simulink model "bikesim_magic_formula"  (R2026a)
settings: Solver=ode45  MaxStep=1E-03
InitFcn:
  | moto_init;
values from neighbouring files (symbols this model uses):
  p = motoParameters    [bikeSimToMotoParameters.m]    (also in moto_init.m = bikeSimToPrydeV2Parameters(bs,130/3.6); moto_trim_test.m = P{idx_vx}; steadyTurningTrimEqns.m = in3(41,:); steadyTurningTrimJac.m = in3(41,:))
  pr = table2struct(rt.Pacejka)    [moto_init.m]    (also in moto_trim_test.m = fpacejka(bs.RearTire.Pacejka))
libraries: simulink x2, simulink_extras x1
(part 1 of 2)
settings Model: Creator=marti  LastModifiedBy=marti

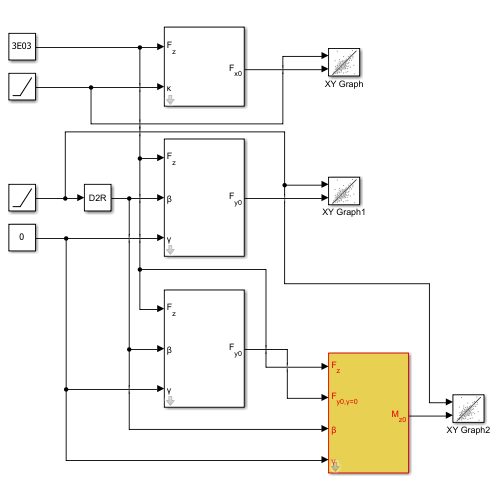
[thumbnail: Simulink's stored preview of the top-level diagram]
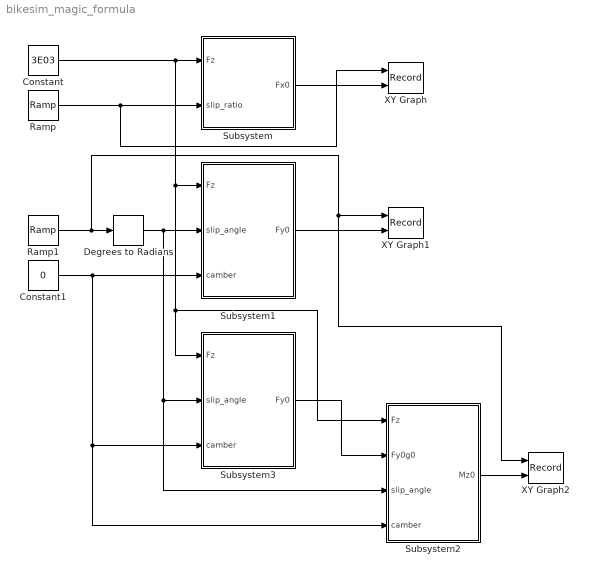
== system bikesim_magic_formula ==
  Constant : Constant  Value=3E03
  Constant1 : Constant  Value=0
  Degrees to Radians : simulink_extras/Transformations/Degrees to Radians
  Ramp : simulink/Sources/Ramp  slope=0.18  start=0  InitialOutput=-0.9
  Ramp1 : simulink/Sources/Ramp  slope=6  start=0  InitialOutput=-30
  Subsystem : Subsystem  mask(Longitudinal force (pure slip)){Fz0=pr.fz0, Cx=pr.pcx1, pdx1=pr.pdx1, pdx2=pr.pdx2, pex1=pr.pex1, pex2=pr.pex2, pex3=pr.pex3, pkx1=pr.pkx1, pkx2=pr.pkx2, pkx3=pr.pkx3}
      mask prompts: Fz0 "F_z0"; Cx "C_x"; pdx1 "p_Dx1"; pdx2 "p_Dx2"; pex1 "p_Ex1"; pex2 "p_Ex2"; pex3 "p_Ex3"; pkx1 "p_Kx1"; pkx2 "p_Kx2"; pkx3 "p_Kx3"
      mask help: Implements (11)-(16) from the BikeSim 2017.1 Tire_Models documentation.
      mask TypeOptions Fz0: Normal force ratio/Fz0
      mask TypeOptions Cx: Magic formula/Cx | Stiffness factor/Cx
      mask TypeOptions pdx1: Peak factor/pdx1
      mask TypeOptions pdx2: Peak factor/pdx2
      mask TypeOptions pex1: Curvature factor/pex1
      mask TypeOptions pex2: Curvature factor/pex2
      mask TypeOptions pex3: Curvature factor/pex3
      mask TypeOptions pkx1: Stiffness factor/pkx1
      mask TypeOptions pkx2: Stiffness factor/pkx2
      mask TypeOptions pkx3: Stiffness factor/pkx3
      mask Display:
      | port_label('input', 1, 'F_z','Interpreter','tex');
      | port_label('input', 2, '\kappa','Interpreter','tex');
      | port_label('output', 1, 'F_{x0}','Interpreter','tex');
  Subsystem1 : Subsystem  mask{Fz0=pr.fz0, Cy=pr.pcy1, Cg=pr.pcy2, pdy1=pr.pdy1, pdy2=pr.pdy2, pdy3=pr.pdy3, pey1=pr.pey1, pey2=pr.pey2, pey4=pr.pey4, Eg=pr.pey5, pky1=pr.pky1, pky2=pr.pky2, pky3=pr.pky3, pky4=pr.pky4, pky5=pr.pky5, pky6=pr.pky6, pky7=pr.pky7}
      mask prompts: Fz0 "F_z0"; Cy "C_y"; Cg "C_g"; pdy1 "p_Dy1"; pdy2 "p_Dy2"; pdy3 "p_Dy3"; pey1 "p_Ey1"; pey2 "p_Ey2"; pey4 "p_Ey4"; Eg "E_g"; pky1 "p_Ky1"; pky2 "p_Ky2"; pky3 "p_Ky3"; pky4 "p_Ky4"; pky5 "p_Ky5"; pky6 "p_Ky6"; pky7 "p_Ky7"
      mask TypeOptions Fz0: Normal force ratio/Fz0 | Lateral force (slip)/Fz0
      mask TypeOptions Cy: Lateral force (slip)/Cy
      mask TypeOptions Cg: Lateral force (camber)/Cg
      mask TypeOptions pdy1: Peak factor/pdy1
      mask TypeOptions pdy2: Peak factor/pdy2
      mask TypeOptions pdy3: Peak factor/pdy3
      mask TypeOptions pey1: Lateral force (slip)/pey1
      mask TypeOptions pey2: Lateral force (slip)/pey2
      mask TypeOptions pey4: Lateral force (slip)/pey4
      mask TypeOptions Eg: Lateral force (camber)/Eg
      mask TypeOptions pky1: Lateral force (slip)/pky1
      mask TypeOptions pky2: Lateral force (slip)/pky2
      mask TypeOptions pky3: Lateral force (slip)/pky3
      mask TypeOptions pky4: Lateral force (slip)/pky4
      mask TypeOptions pky5: Lateral force (slip)/pky5
      mask TypeOptions pky6: Lateral force (camber)/pky6
      mask TypeOptions pky7: Lateral force (camber)/pky7
      mask Display:
      | port_label('input', 1, 'F_z','Interpreter','tex');
      | port_label('input', 2, '\beta','Interpreter','tex');
      | port_label('input', 3, '\gamma','Interpreter','tex');
      | port_label('output', 1, 'F_{y0}','Interpreter','tex');
  Subsystem2 : Subsystem  mask{R0=p.tr, Cy=pr.pcy1, Ct=pr.qcz1, Fz0=pr.fz0, qbz1=pr.qbz1, qbz2=pr.qbz2, qbz5=pr.qbz5, qbz6=pr.qbz6, qbz9=pr.qbz9, qbz10=pr.qbz10, qdz1=pr.qdz1, qdz2=pr.qdz2, qdz3=pr.qdz3, qdz4=pr.qdz4, qdz8=pr.qdz8, qdz9=pr.qdz9, qdz10=pr.qdz10, qdz11=pr.qdz11, qez1=pr.qez1, qez2=pr.qez2, qez5=pr.qez5, qhz3=pr.qhz3, qhz4=pr.qhz4}
      mask prompts: R0 "R_0"; Cy "C_y"; Ct "C_t"; Fz0 "F_z0"; qbz1 "q_Bz1"; qbz2 "q_Bz2"; qbz5 "q_Bz5"; qbz6 "q_Bz6"; qbz9 "q_Bz9"; qbz10 "q_Bz10"; qdz1 "q_Dz1"; qdz2 "q_Dz2"; qdz3 "q_Dz3"; qdz4 "q_Dz4"; qdz8 "q_Dz8"; qdz9 "q_Dz9"; qdz10 "q_Dz10"; qdz11 "q_Dz11"; qez1 "q_Ez1"; qez2 "q_Ez2"; qez5 "q_Ez5"; qhz3 "q_Hz3"; qhz4 "q_Hz4"
      mask TypeOptions R0: Aligning moment (residual)/R0 | Aligning moment (trail)/R0
      mask TypeOptions Cy: Aligning moment (residual)/Cy
      mask TypeOptions Ct: Aligning moment (trail)/Ct
      mask TypeOptions Fz0: Aligning moment (trail)/Fz0
      mask TypeOptions qbz1: Aligning moment (trail)/qbz1
      mask TypeOptions qbz2: Aligning moment (trail)/qbz2
      mask TypeOptions qbz5: Aligning moment (trail)/qbz5
      mask TypeOptions qbz6: Aligning moment (trail)/qbz6
      mask TypeOptions qbz9: Aligning moment (residual)/qbz9
      mask TypeOptions qbz10: Aligning moment (residual)/qbz10
      mask TypeOptions qdz1: Aligning moment (trail)/qdz1
      mask TypeOptions qdz2: Aligning moment (trail)/qdz2
      mask TypeOptions qdz3: Aligning moment (trail)/qdz3
      mask TypeOptions qdz4: Aligning moment (trail)/qdz4
      mask TypeOptions qdz8: Aligning moment (residual)/qdz8
      mask TypeOptions qdz9: Aligning moment (residual)/qdz9
      mask TypeOptions qdz10: Aligning moment (residual)/qdz10
      mask TypeOptions qdz11: Aligning moment (residual)/qdz11
      mask TypeOptions qez1: Aligning moment (trail)/qez1
      mask TypeOptions qez2: Aligning moment (trail)/qez2
      mask TypeOptions qez5: Aligning moment (trail)/qez5
      mask TypeOptions qhz3: Aligning moment (residual)/qhz3
      mask TypeOptions qhz4: Aligning moment (residual)/qhz4
      mask Display:
      | port_label('input', 1, 'F_z','Interpreter','tex');
      | port_label('input', 2, 'F_{y0,\gamma=0}','Interpreter','tex');
      | port_label('input', 3, '\beta','Interpreter','tex');
      | port_label('input', 4, '\gamma','Interpreter','tex');
      | port_label('output', 1, 'M_{z0}','Interpreter','tex');
  Subsystem3 : Subsystem  mask{Fz0=pr.fz0, Cy=pr.pcy1, Cg=pr.pcy2, pdy1=pr.pdy1, pdy2=pr.pdy2, pdy3=pr.pdy3, pey1=pr.pey1, pey2=pr.pey2, pey4=pr.pey4, Eg=pr.pey5, pky1=pr.pky1, pky2=pr.pky2, pky3=pr.pky3, pky4=pr.pky4, pky5=pr.pky5, pky6=pr.pky6, pky7=pr.pky7}
      mask prompts: Fz0 "F_z0"; Cy "C_y"; Cg "C_g"; pdy1 "p_Dy1"; pdy2 "p_Dy2"; pdy3 "p_Dy3"; pey1 "p_Ey1"; pey2 "p_Ey2"; pey4 "p_Ey4"; Eg "E_g"; pky1 "p_Ky1"; pky2 "p_Ky2"; pky3 "p_Ky3"; pky4 "p_Ky4"; pky5 "p_Ky5"; pky6 "p_Ky6"; pky7 "p_Ky7"
      mask TypeOptions Fz0: Normal force ratio/Fz0 | Lateral force (slip)/Fz0
      mask TypeOptions Cy: Lateral force (slip)/Cy
      mask TypeOptions Cg: Lateral force (camber)/Cg
      mask TypeOptions pdy1: Peak factor/pdy1
      mask TypeOptions pdy2: Peak factor/pdy2
      mask TypeOptions pdy3: Peak factor/pdy3
      mask TypeOptions pey1: Lateral force (slip)/pey1
      mask TypeOptions pey2: Lateral force (slip)/pey2
      mask TypeOptions pey4: Lateral force (slip)/pey4
      mask TypeOptions Eg: Lateral force (camber)/Eg
      mask TypeOptions pky1: Lateral force (slip)/pky1
      mask TypeOptions pky2: Lateral force (slip)/pky2
      mask TypeOptions pky3: Lateral force (slip)/pky3
      mask TypeOptions pky4: Lateral force (slip)/pky4
      mask TypeOptions pky5: Lateral force (slip)/pky5
      mask TypeOptions pky6: Lateral force (camber)/pky6
      mask TypeOptions pky7: Lateral force (camber)/pky7
      mask Display:
      | port_label('input', 1, 'F_z','Interpreter','tex');
      | port_label('input', 2, '\beta','Interpreter','tex');
      | port_label('input', 3, '\gamma','Interpreter','tex');
      | port_label('output', 1, 'F_{y0}','Interpreter','tex');
  XY Graph : Record  NumPorts=2.0  FileSettingsInternal="{\"entries\":[{\"content\":{\"excelSettings\":{\"content\":{},\"type\":\"Streamout.ExcelSettings\"},\"parquetSettings\":{\"content\":{},\"type\":\"Streamout.ParquetSettings\"}},\"type\":\"Streamout.FileSettingStorage\",\"uuid\":\"\"}],\"packageUris\":[\"http:\\/\\/schema.mathworks.com\\/mf0\\/streamout_blocks\\/R2020a\"],\"version\":\"1.0\"}"  FrameSettings=[0, 0]  Layout=[1 1]  SignalsInternal="{\"entries\":[{\"content\":{\"signals\":[{\"content\":{\"blockPath\":[],\"dimensions\":[1],\"domain\":\"\",\"lineColor\":\"#a2142f\",\"plots\":[ 1 ],\"port\":1,\"sid\":[\"\"],\"signalID\":1,\"signalName\":\"Ramp\"},\"type\":\"RecordBlkView.Signal\",\"uuid\":\"\"},{\"content\":{\"blockPath\":[],\"dimensions\":[1],\"domain\":\"\",\"lineColor\":\"#139fff\",\"plots\":[ 1 ],\"port\":2,\"sid\":[\"\"],\"signalID\":2,\"signalName\":\"Subsystem\"},\"type\":\"RecordBlkView.Signal\",\"uuid\":\"\"}]},\"type\":\"RecordBlkView.InputSignals\",\"uuid\":\"\"}],\"packageUris\":[\"http:\\/\\/schema.mathworks.com\\/mf0\\/streamout_blocks\\/R2020a\"],\"version\":\"1.0\"}"  VisualizationBindings="{\"xyplotplugin\":{\"info\":[{\"series\":[{\"bindingParametersList\":[{\"parameter\":\"X-Axis\",\"signalID\":1,\"signalName\":\"Ramp\"},{\"parameter\":\"Y-Axis\",\"signalID\":2,\"signalName\":\"Subsystem\"}],\"seriesID\":0}],\"subplotID\":1}]}}"  CompatibilityTag=XY
  XY Graph1 : Record  NumPorts=2.0  FileSettingsInternal="{\"entries\":[{\"content\":{\"excelSettings\":{\"content\":{},\"type\":\"Streamout.ExcelSettings\"},\"parquetSettings\":{\"content\":{},\"type\":\"Streamout.ParquetSettings\"}},\"type\":\"Streamout.FileSettingStorage\",\"uuid\":\"\"}],\"packageUris\":[\"http:\\/\\/schema.mathworks.com\\/mf0\\/streamout_blocks\\/R2020a\"],\"version\":\"1.0\"}"  FrameSettings=[0, 0]  Layout=[1 1]  SignalsInternal="{\"entries\":[{\"content\":{\"signals\":[{\"content\":{\"blockPath\":[],\"dimensions\":[1],\"domain\":\"\",\"lineColor\":\"#a2142f\",\"plots\":[ 1 ],\"port\":1,\"sid\":[\"\"],\"signalID\":1,\"signalName\":\"Ramp1\"},\"type\":\"RecordBlkView.Signal\",\"uuid\":\"\"},{\"content\":{\"blockPath\":[],\"dimensions\":[1],\"domain\":\"\",\"lineColor\":\"#139fff\",\"plots\":[ 1 ],\"port\":2,\"sid\":[\"\"],\"signalID\":2,\"signalName\":\"Subsystem1\"},\"type\":\"RecordBlkView.Signal\",\"uuid\":\"\"}]},\"type\":\"RecordBlkView.InputSignals\",\"uuid\":\"\"}],\"packageUris\":[\"http:\\/\\/schema.mathworks.com\\/mf0\\/streamout_blocks\\/R2020a\"],\"version\":\"1.0\"}"  VisualizationBindings="{\"xyplotplugin\":{\"info\":[{\"series\":[{\"bindingParametersList\":[{\"parameter\":\"X-Axis\",\"signalID\":1,\"signalName\":\"Ramp1\"},{\"parameter\":\"Y-Axis\",\"signalID\":2,\"signalName\":\"Subsystem1\"}],\"seriesID\":0}],\"subplotID\":1}]}}"  CompatibilityTag=XY
  XY Graph2 : Record  NumPorts=2.0  FileSettingsInternal="{\"entries\":[{\"content\":{\"excelSettings\":{\"content\":{},\"type\":\"Streamout.ExcelSettings\"},\"parquetSettings\":{\"content\":{},\"type\":\"Streamout.ParquetSettings\"}},\"type\":\"Streamout.FileSettingStorage\",\"uuid\":\"\"}],\"packageUris\":[\"http:\\/\\/schema.mathworks.com\\/mf0\\/streamout_blocks\\/R2020a\"],\"version\":\"1.0\"}"  FrameSettings=[0, 0]  Layout=[1 1]  SignalsInternal="{\"entries\":[{\"content\":{\"signals\":[{\"content\":{\"blockPath\":[],\"dimensions\":[1],\"domain\":\"\",\"lineColor\":\"#a2142f\",\"plots\":[ 1 ],\"port\":1,\"signalID\":1,\"signalName\":\"XY Graph:1\"},\"type\":\"RecordBlkView.Signal\",\"uuid\":\"\"},{\"content\":{\"blockPath\":[],\"dimensions\":[1],\"domain\":\"\",\"lineColor\":\"#139fff\",\"plots\":[ 1 ],\"port\":2,\"signalID\":2,\"signalName\":\"XY Graph:2\"},\"type\":\"RecordBlkView.Signal\",\"uuid\":\"\"}]},\"type\":\"RecordBlkView.InputSignals\",\"uuid\":\"\"}],\"packageUris\":[\"http:\\/\\/schema.mathworks.com\\/mf0\\/streamout_blocks\\/R2020a\"],\"version\":\"1.0\"}"  VisualizationBindings="{\"xyplotplugin\":{\"info\":[{\"series\":[{\"bindingParametersList\":[{\"parameter\":\"X-Axis\",\"signalID\":1,\"signalName\":\"XY Graph:1\"},{\"parameter\":\"Y-Axis\",\"signalID\":2,\"signalName\":\"XY Graph:2\"}],\"seriesID\":0}],\"subplotID\":1}]}}"  CompatibilityTag=XY
  wires:
  Constant/1 -> Subsystem3/1(Fz), Subsystem2/1(Fz), Subsystem1/1(Fz), Subsystem/1(Fz)
  Ramp/1 -> XY Graph/1, Subsystem/2(slip_ratio)
  Ramp1/1 -> XY Graph2/1, XY Graph1/1, Degrees to Radians/1
  Constant1/1 -> Subsystem2/4(camber), Subsystem3/3(camber), Subsystem1/3(camber)
  Degrees to Radians/1 -> Subsystem2/3(slip_angle), Subsystem3/2(slip_angle), Subsystem1/2(slip_angle)
  Subsystem/1(Fx0) -> XY Graph/2
  Subsystem1/1(Fy0) -> XY Graph1/2
  Subsystem3/1(Fy0) -> Subsystem2/2(Fy0g0)
  Subsystem2/1(Mz0) -> XY Graph2/2

== system bikesim_magic_formula/Subsystem ==
  Fz : Inport
  slip_ratio : Inport  Port=2
  Curvature factor : Subsystem  mask(Curvature factor: longitudinal){pex1=pex1, pex2=pex2, pex3=pex3}
      mask prompts: pex1 "p_Ex1"; pex2 "p_Ex2"; pex3 "p_Ex3"
      mask help: Implements (14) from the BikeSim 2017.1 Tire_Models documentation.
      mask Display:
      | port_label('input', 1, 'd_{fz}','Interpreter','tex');
      | port_label('input', 2, '\kappa','Interpreter','tex');
      | port_label('output', 1, 'E_x','Interpreter','tex');
      | disp('(p_{Ex1} + p_{Ex2}\cdotdf_z + p_{Ex3}\cdotdf_{z}^{2})\cdot(1 - sgn(\kappa))','Interpreter','tex');
  Magic formula : Subsystem  mask(Magic formula: longitudinal (pure slip)){Cx=Cx}
      mask prompts: Cx "C_x"
      mask help: Implements (12) from the BikeSim 2017.1 Tire_Models documentation.
      mask TypeOptions Cx: Cx/Gain
      mask Display:
      | port_label('input', 1, 'D_x','Interpreter','tex');
      | port_label('input', 2, 'E_x','Interpreter','tex');
      | port_label('input', 3, 'B_x','Interpreter','tex');
      | port_label('input', 4, '\kappa','Interpreter','tex');
      | port_label('output', 1, 'F_{x0}','Interpreter','tex');
      | disp('D_x\cdotsin(C_x\cdotatan(B_x\cdot\kappa - E_x\cdot(B_x\cdot\kappa - atan(B_x\cdot\kappa))))','Interpreter','tex');
  Normal force ratio : Subsystem  mask(Normal force ratio){Fz0=Fz0}
      mask prompts: Fz0 "Nominal normal force"
      mask help: Implements (11) from the BikeSim 2017.1 Tire_models help documentation.
      mask TypeOptions Fz0: Fz0/Value
      mask Display:
      | port_label('output', 1, 'df_z','interpreter','tex');
      | port_label('input', 1, 'F_z','interpreter','tex');
      | disp('(F_z - F_{z0})/F_{z0}','interpreter','tex');
  Peak factor : Subsystem  mask(Peak factor: longitudinal){pdx1=pdx1, pdx2=pdx2}
      mask prompts: pdx1 "p_Dx1"; pdx2 "p_Dx2"
      mask help: Implements (13) from the BikeSim 2017.1 Tire_Models documentation.
      mask Display:
      | port_label('input', 1, 'F_z','Interpreter','tex');
      | port_label('input', 2, 'df_z','Interpreter','tex');
      | port_label('output', 1, 'D_x','Interpreter','tex');
      | disp('(p_{Dx1} + p_{Dx2}\cdotdf_z)\cdotF_z','Interpreter','tex');
  Stiffness factor : Subsystem  mask(Stiffness factor: longitudinal){pkx1=pkx1, pkx2=pkx2, pkx3=pkx3, Cx=Cx}
      mask prompts: pkx1 "p_Kx1"; pkx2 "p_Kx2"; pkx3 "p_Kx3"; Cx "C_x"
      mask help: Implements (15) and (16) from the BikeSim 2017.1 Tire_Models documentation.
      mask TypeOptions Cx: Cx/Gain
      mask Display:
      | port_label('input', 1, 'F_z','Interpreter','tex');
      | port_label('input', 2, 'df_z','Interpreter','tex');
      | port_label('input', 3, 'D_x','Interpreter','tex');
      | port_label('output', 1, 'B_x','Interpreter','tex');
      | disp('(F_z\cdot(p_{Kx1} + p_{Kx2}\cdotdf_z)\cdote^{(p_{Kx3}\cdotdf_z)})/(C_x\cdotD_x)','Interpreter','tex');
  Fx0 : Outport
  wires:
  Normal force ratio/1(dfz) -> Curvature factor/1(dfz), Stiffness factor/2(dfz), Peak factor/2(dfz)
  Fz/1 -> Stiffness factor/1(Fz), Peak factor/1(Fz), Normal force ratio/1(Fz)
  Peak factor/1(Dx) -> Magic formula/1(Dx), Stiffness factor/3(Dx)
  slip_ratio/1 -> Magic formula/4(slip_ratio), Curvature factor/2(slip_ratio)
  Curvature factor/1(Ex) -> Magic formula/2(Ex)
  Stiffness factor/1(Bx) -> Magic formula/3(Bx)
  Magic formula/1(Fx0) -> Fx0/1

== system bikesim_magic_formula/Subsystem1 ==
  Fz : Inport
  slip_angle : Inport  Port=2
  camber : Inport  Port=3
  Lateral force (camber) : Subsystem  mask{Cg=Cg, Eg=Eg, pky6=pky6, pky7=pky7}
      mask prompts: Cg "C_g"; Eg "E_g"; pky6 "p_Ky6"; pky7 "p_Ky7"
      mask TypeOptions Cg: Cg/Gain | Stiffness factor/Cg
      mask TypeOptions Eg: Eg/Gain
      mask TypeOptions pky6: Stiffness factor/pky6
      mask TypeOptions pky7: Stiffness factor/pky7
      mask Display:
      | port_label('input', 1, 'F_z','Interpreter','tex');
      | port_label('input', 2, 'df_z','Interpreter','tex');
      | port_label('input', 3, '\gamma','Interpreter','tex');
      | port_label('input', 4, 'D_y','Interpreter','tex');
      | port_label('output', 1, 'F_{y0\gamma}','Interpreter','tex');
  Lateral force (slip) : Subsystem  mask{Fz0=Fz0, Cy=Cy, pey1=pey1, pey2=pey2, pey4=pey4, pky1=pky1, pky2=pky2, pky3=pky3, pky4=pky4, pky5=pky5}
      mask prompts: Fz0 "F_z0"; Cy "C_y"; pey1 "p_Ey1"; pey2 "p_Ey2"; pey4 "p_Ey4"; pky1 "p_Ky1"; pky2 "p_Ky2"; pky3 "p_Ky3"; pky4 "p_Ky4"; pky5 "p_Ky5"
      mask TypeOptions Fz0: Stiffness factor/Fz0
      mask TypeOptions Cy: Cy/Gain | Stiffness factor/Cy
      mask TypeOptions pey1: Curvature factor/pey1
      mask TypeOptions pey2: Curvature factor/pey2
      mask TypeOptions pey4: Curvature factor/pey4
      mask TypeOptions pky1: Stiffness factor/pky1
      mask TypeOptions pky2: Stiffness factor/pky2
      mask TypeOptions pky3: Stiffness factor/pky3
      mask TypeOptions pky4: Stiffness factor/pky4
      mask TypeOptions pky5: Stiffness factor/pky5
      mask Display:
      | port_label('input', 1, 'F_z','Interpreter','tex');
      | port_label('input', 2, '\beta','Interpreter','tex');
      | port_label('input', 3, '\gamma','Interpreter','tex');
      | port_label('input', 4, 'D_y','Interpreter','tex');
      | port_label('output', 1, 'F_{y0\beta}','Interpreter','tex');
  Normal force ratio : Subsystem  mask(Normal force ratio){Fz0=Fz0}
      mask prompts: Fz0 "Nominal normal force"
      mask help: Implements (11) from the BikeSim 2017.1 Tire_models help documentation.
      mask TypeOptions Fz0: Fz0/Value
      mask Display:
      | port_label('output', 1, 'df_z','interpreter','tex');
      | port_label('input', 1, 'F_z','interpreter','tex');
      | disp('(F_z - F_{z0})/F_{z0}','interpreter','tex');
  Peak factor : Subsystem  mask{pdy1=pdy1, pdy2=pdy2, pdy3=pdy3}
      mask prompts: pdy1 "p_Dy1"; pdy2 "p_Dy2"; pdy3 "p_Dy3"
      mask TypeOptions pdy1: pdy1/Gain
      mask TypeOptions pdy2: pdy2/Gain
      mask Display:
      | port_label('input', 1, 'F_z','Interpreter','tex');
      | port_label('input', 2, 'df_z','Interpreter','tex');
      | port_label('input', 3, '\gamma','Interpreter','tex');
      | port_label('output', 1, 'D_y','Interpreter','tex');
  Product : Product
  Sin : Trigonometry
  Sum : Sum  Inputs=|++
  Fy0 : Outport
  wires:
  Fz/1 -> Lateral force (slip)/1(Fz), Lateral force (camber)/1(Fz), Peak factor/1(Fz), Normal force ratio/1(Fz)
  Normal force ratio/1(dfz) -> Lateral force (camber)/2(dfz), Peak factor/2(dfz)
  camber/1 -> Lateral force (camber)/3(camber), Lateral force (slip)/3(camber), Peak factor/3(camber)
  slip_angle/1 -> Lateral force (slip)/2(slip_angle)
  Peak factor/1(Dy) -> Product/1, Lateral force (camber)/4(Dy), Lateral force (slip)/4(Dy)
  Lateral force (slip)/1(Fy0a) -> Sum/1
  Lateral force (camber)/1(Fy0g) -> Sum/2
  Sum/1 -> Sin/1
  Sin/1 -> Product/2
  Product/1 -> Fy0/1

== system bikesim_magic_formula/Subsystem2 ==
  Fz : Inport
  Fy0g0 : Inport  Port=2
  slip_angle : Inport  Port=3
  camber : Inport  Port=4
  Aligning moment (residual) : Subsystem  mask{R0=R0, Cy=Cy, qbz9=qbz9, qbz10=qbz10, qdz8=qdz8, qdz9=qdz9, qdz10=qdz10, qdz11=qdz11, qhz3=qhz3, qhz4=qhz4}
      mask prompts: R0 "R_0"; Cy "C_y"; qbz9 "q_Bz9"; qbz10 "q_Bz10"; qdz8 "q_Dz8"; qdz9 "q_Dz9"; qdz10 "q_Dz10"; qdz11 "q_Dz11"; qhz3 "q_Hz3"; qhz4 "q_Hz4"
      mask TypeOptions R0: Peak factor/R0
      mask TypeOptions Cy: Stiffness factor/Cy
      mask TypeOptions qbz9: Stiffness factor/qbz9
      mask TypeOptions qbz10: Stiffness factor/qbz10
      mask TypeOptions qdz8: Peak factor/qdz8
      mask TypeOptions qdz9: Peak factor/qdz9
      mask TypeOptions qdz10: Peak factor/qdz10
      mask TypeOptions qdz11: Peak factor/qdz11
      mask TypeOptions qhz3: Horizontal shift/qhz3
      mask TypeOptions qhz4: Horizontal shift/qhz4
      mask Display:
      | port_label('input', 1, 'F_z','Interpreter','tex');
      | port_label('input', 2, 'df_z','Interpreter','tex');
      | port_label('input', 3, 'B_y','Interpreter','tex');
      | port_label('input', 4, '\beta','Interpreter','tex');
      | port_label('input', 5, '\gamma','Interpreter','tex');
      | port_label('output', 1, 'M_{zr0}','Interpreter','tex');
  Aligning moment (trail) : Subsystem  mask{R0=R0, Ct=Ct, Fz0=Fz0, qbz1=qbz1, qbz2=qbz2, qbz5=qbz5, qbz6=qbz6, qdz1=qdz1, qdz2=qdz2, qdz3=qdz3, qdz4=qdz4, qez1=qez1, qez2=qez2, qez5=qez5}
      mask prompts: R0 "R_0"; Ct "C_t"; Fz0 "F_z0"; qbz1 "q_Bz1"; qbz2 "q_Bz2"; qbz5 "q_Bz5"; qbz6 "q_Bz6"; qdz1 "q_Dz1"; qdz2 "q_Dz2"; qdz3 "q_Dz3"; qdz4 "q_Dz4"; qez1 "q_Ez1"; qez2 "q_Ez2"; qez5 "q_Ez5"
      mask TypeOptions R0: Peak factor/R0
      mask TypeOptions Ct: Ct/Gain | Curvature factor/Ct
      mask TypeOptions Fz0: Peak factor/Fz0
      mask TypeOptions qbz1: Stiffness factor/qbz1
      mask TypeOptions qbz2: Stiffness factor/qbz2
      mask TypeOptions qbz5: Stiffness factor/qbz5
      mask TypeOptions qbz6: Stiffness factor/qbz6
      mask TypeOptions qdz1: Peak factor/qdz1
      mask TypeOptions qdz2: Peak factor/qdz2
      mask TypeOptions qdz3: Peak factor/qdz3
      mask TypeOptions qdz4: Peak factor/qdz4
      mask TypeOptions qez1: Curvature factor/qez1
      mask TypeOptions qez2: Curvature factor/qez2
      mask TypeOptions qez5: Curvature factor/qez5
      mask Display:
      | port_label('input', 1, 'F_z','Interpreter','tex');
      | port_label('input', 2, 'df_z','Interpreter','tex');
      | port_label('input', 3, '\beta','Interpreter','tex');
      | port_label('input', 4, '\gamma','Interpreter','tex');
      | port_label('input', 5, 'F_{y0,\gamma=0}','Interpreter','tex');
      | port_label('output', 1, 'M_{zt0}','Interpreter','tex');
  Normal force ratio : Subsystem  mask(Normal force ratio){Fz0=1}
      mask prompts: Fz0 "Nominal normal force"
      mask help: Implements (11) from the BikeSim 2017.1 Tire_models help documentation.
      mask TypeOptions Fz0: Fz0/Value
      mask Display:
      | port_label('output', 1, 'df_z','interpreter','tex');
      | port_label('input', 1, 'F_z','interpreter','tex');
      | disp('(F_z - F_{z0})/F_{z0}','interpreter','tex');
  Peak factor : Subsystem  mask{pdy1=0, pdy2=0, pdy3=0}
      mask prompts: pdy1 "p_Dy1"; pdy2 "p_Dy2"; pdy3 "p_Dy3"
      mask TypeOptions pdy1: pdy1/Gain
      mask TypeOptions pdy2: pdy2/Gain
      mask Display:
      | port_label('input', 1, 'F_z','Interpreter','tex');
      | port_label('input', 2, 'df_z','Interpreter','tex');
      | port_label('input', 3, '\gamma','Interpreter','tex');
      | port_label('output', 1, 'D_y','Interpreter','tex');
  Stiffness factor : Subsystem  mask{Fz0=0, Cy=0, pky1=0, pky2=0, pky3=0, pky4=0, pky5=0}
      mask prompts: Fz0 "F_z0"; Cy "C_y"; pky1 "p_Ky1"; pky2 "p_Ky2"; pky3 "p_Ky3"; pky4 "p_Ky4"; pky5 "p_Ky5"
      mask TypeOptions Fz0: Fz0/Gain | Fz01/Gain
      mask TypeOptions Cy: Cy/Gain
      mask TypeOptions pky1: pky1/Gain
      mask TypeOptions pky2: pky2/Gain
      mask Display:
      | port_label('input', 1, 'F_z','Interpreter','tex');
      | port_label('input', 2, '\gamma','Interpreter','tex');
      | port_label('input', 3, 'D_y','Interpreter','tex');
      | port_label('output', 1, 'B_y','Interpreter','tex');
  Sum : Sum  Inputs=|++
  Mz0 : Outport
  wires:
  Peak factor/1(Dy) -> Stiffness factor/3(Dy)
  Normal force ratio/1(dfz) -> Peak factor/2(dfz), Aligning moment (residual)/2(dfz), Aligning moment (trail)/2(dfz)
  Fz/1 -> Aligning moment (trail)/1(Fz), Normal force ratio/1(Fz), Aligning moment (residual)/1(Fz), Stiffness factor/1(Fz), Peak factor/1(Fz)
  camber/1 -> Aligning moment (trail)/4(camber), Stiffness factor/2(camber), Peak factor/3(camber), Aligning moment (residual)/5(camber)
  Stiffness factor/1(By) -> Aligning moment (residual)/3(By)
  slip_angle/1 -> Aligning moment (residual)/4(slip_angle), Aligning moment (trail)/3(slip_angle)
  Fy0g0/1 -> Aligning moment (trail)/5(Fy0g0)
  Aligning moment (residual)/1(Mzr0) -> Sum/1
  Aligning moment (trail)/1(Mzt0) -> Sum/2
  Sum/1 -> Mz0/1

== system bikesim_magic_formula/Subsystem3 ==
  Fz : Inport
  slip_angle : Inport  Port=2
  camber : Inport  Port=3
  Lateral force (camber) : Subsystem  mask{Cg=Cg, Eg=Eg, pky6=pky6, pky7=pky7}
      mask prompts: Cg "C_g"; Eg "E_g"; pky6 "p_Ky6"; pky7 "p_Ky7"
      mask TypeOptions Cg: Cg/Gain | Stiffness factor/Cg
      mask TypeOptions Eg: Eg/Gain
      mask TypeOptions pky6: Stiffness factor/pky6
      mask TypeOptions pky7: Stiffness factor/pky7
      mask Display:
      | port_label('input', 1, 'F_z','Interpreter','tex');
      | port_label('input', 2, 'df_z','Interpreter','tex');
      | port_label('input', 3, '\gamma','Interpreter','tex');
      | port_label('input', 4, 'D_y','Interpreter','tex');
      | port_label('output', 1, 'F_{y0\gamma}','Interpreter','tex');
  Lateral force (slip) : Subsystem  mask{Fz0=Fz0, Cy=Cy, pey1=pey1, pey2=pey2, pey4=pey4, pky1=pky1, pky2=pky2, pky3=pky3, pky4=pky4, pky5=pky5}
      mask prompts: Fz0 "F_z0"; Cy "C_y"; pey1 "p_Ey1"; pey2 "p_Ey2"; pey4 "p_Ey4"; pky1 "p_Ky1"; pky2 "p_Ky2"; pky3 "p_Ky3"; pky4 "p_Ky4"; pky5 "p_Ky5"
      mask TypeOptions Fz0: Stiffness factor/Fz0
      mask TypeOptions Cy: Cy/Gain | Stiffness factor/Cy
      mask TypeOptions pey1: Curvature factor/pey1
      mask TypeOptions pey2: Curvature factor/pey2
      mask TypeOptions pey4: Curvature factor/pey4
      mask TypeOptions pky1: Stiffness factor/pky1
      mask TypeOptions pky2: Stiffness factor/pky2
      mask TypeOptions pky3: Stiffness factor/pky3
      mask TypeOptions pky4: Stiffness factor/pky4
      mask TypeOptions pky5: Stiffness factor/pky5
      mask Display:
      | port_label('input', 1, 'F_z','Interpreter','tex');
      | port_label('input', 2, '\beta','Interpreter','tex');
      | port_label('input', 3, '\gamma','Interpreter','tex');
      | port_label('input', 4, 'D_y','Interpreter','tex');
      | port_label('output', 1, 'F_{y0\beta}','Interpreter','tex');
  Normal force ratio : Subsystem  mask(Normal force ratio){Fz0=Fz0}
      mask prompts: Fz0 "Nominal normal force"
      mask help: Implements (11) from the BikeSim 2017.1 Tire_models help documentation.
      mask TypeOptions Fz0: Fz0/Value
      mask Display:
      | port_label('output', 1, 'df_z','interpreter','tex');
      | port_label('input', 1, 'F_z','interpreter','tex');
      | disp('(F_z - F_{z0})/F_{z0}','interpreter','tex');
  Peak factor : Subsystem  mask{pdy1=pdy1, pdy2=pdy2, pdy3=pdy3}
      mask prompts: pdy1 "p_Dy1"; pdy2 "p_Dy2"; pdy3 "p_Dy3"
      mask TypeOptions pdy1: pdy1/Gain
      mask TypeOptions pdy2: pdy2/Gain
      mask Display:
      | port_label('input', 1, 'F_z','Interpreter','tex');
      | port_label('input', 2, 'df_z','Interpreter','tex');
      | port_label('input', 3, '\gamma','Interpreter','tex');
      | port_label('output', 1, 'D_y','Interpreter','tex');
  Product : Product
  Sin : Trigonometry
  Sum : Sum  Inputs=|++
  Fy0 : Outport
  wires:
  Fz/1 -> Lateral force (slip)/1(Fz), Lateral force (camber)/1(Fz), Peak factor/1(Fz), Normal force ratio/1(Fz)
  Normal force ratio/1(dfz) -> Lateral force (camber)/2(dfz), Peak factor/2(dfz)
  camber/1 -> Lateral force (camber)/3(camber), Lateral force (slip)/3(camber), Peak factor/3(camber)
  slip_angle/1 -> Lateral force (slip)/2(slip_angle)
  Peak factor/1(Dy) -> Product/1, Lateral force (camber)/4(Dy), Lateral force (slip)/4(Dy)
  Lateral force (slip)/1(Fy0a) -> Sum/1
  Lateral force (camber)/1(Fy0g) -> Sum/2
  Sum/1 -> Sin/1
  Sin/1 -> Product/2
  Product/1 -> Fy0/1

== system bikesim_magic_formula/Subsystem/Curvature factor ==
  dfz : Inport
  slip_ratio : Inport  Port=2
  Constant : Constant
  Polynomial : Polyval  Coefs=[pex3,pex2,pex1]
  Product : Product
  Sign : Signum
  Sum : Sum  Inputs=|+-
  Ex : Outport
  wires:
  slip_ratio/1 -> Sign/1
  dfz/1 -> Polynomial/1
  Polynomial/1 -> Product/1
  Constant/1 -> Sum/1
  Sum/1 -> Product/2
  Product/1 -> Ex/1
  Sign/1 -> Sum/2

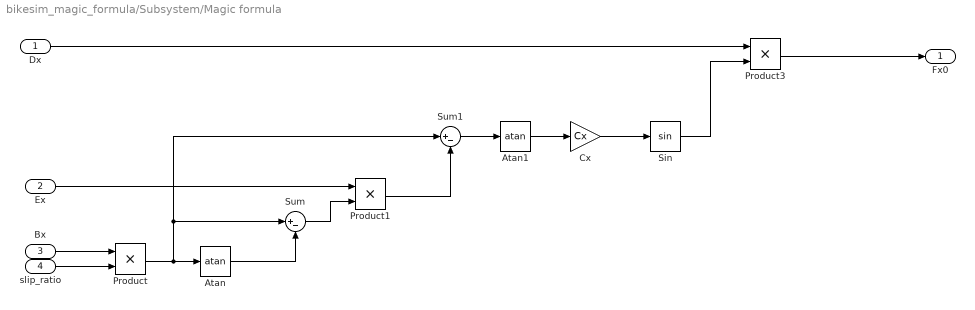
== system bikesim_magic_formula/Subsystem/Magic formula ==
  Dx : Inport
  Ex : Inport  Port=2
  Bx : Inport  Port=3
  slip_ratio : Inport  Port=4
  Atan : Trigonometry  Operator=atan
  Atan1 : Trigonometry  Operator=atan
  Cx : Gain  Gain=Cx
  Product : Product
  Product1 : Product
  Product3 : Product
  Sin : Trigonometry
  Sum : Sum  Inputs=|+-
  Sum1 : Sum  Inputs=|+-
  Fx0 : Outport
  wires:
  Sum1/1 -> Atan1/1
  Product/1 -> Sum1/1, Sum/1, Atan/1
  Product3/1 -> Fx0/1
  Cx/1 -> Sin/1
  Sin/1 -> Product3/2
  Ex/1 -> Product1/1
  Atan/1 -> Sum/2
  Dx/1 -> Product3/1
  Product1/1 -> Sum1/2
  Sum/1 -> Product1/2
  Atan1/1 -> Cx/1
  Bx/1 -> Product/1
  slip_ratio/1 -> Product/2

== system bikesim_magic_formula/Subsystem/Normal force ratio ==
  Fz : Inport
  Divide : Product  Inputs=*/
  Fz0 : Constant  Value=Fz0
  Sum : Sum  Inputs=|+-
  dfz : Outport
  wires:
  Sum/1 -> Divide/1
  Fz0/1 -> Divide/2, Sum/2
  Divide/1 -> dfz/1
  Fz/1 -> Sum/1

== system bikesim_magic_formula/Subsystem/Peak factor ==
  Fz : Inport
  dfz : Inport  Port=2
  Polynomial : Polyval  Coefs=[pdx2,pdx1]
  Product : Product
  Dx : Outport
  wires:
  Polynomial/1 -> Product/2
  Fz/1 -> Product/1
  Product/1 -> Dx/1
  dfz/1 -> Polynomial/1

== system bikesim_magic_formula/Subsystem/Stiffness factor ==
  Fz : Inport
  dfz : Inport  Port=2
  Dx : Inport  Port=3
  Cx : Gain  Gain=Cx
  Divide : Product  Inputs=*/
  Exp : Math
  Polynomial : Polyval  Coefs=[pkx2,pkx1]
  Polynomial1 : Polyval  Coefs=[pkx3,0]
  Product : Product  Inputs=3
  Bx : Outport
  wires:
  dfz/1 -> Polynomial1/1, Polynomial/1
  Dx/1 -> Cx/1
  Cx/1 -> Divide/2
  Polynomial1/1 -> Exp/1
  Polynomial/1 -> Product/2
  Exp/1 -> Product/3
  Product/1 -> Divide/1
  Fz/1 -> Product/1
  Divide/1 -> Bx/1  "Bx"

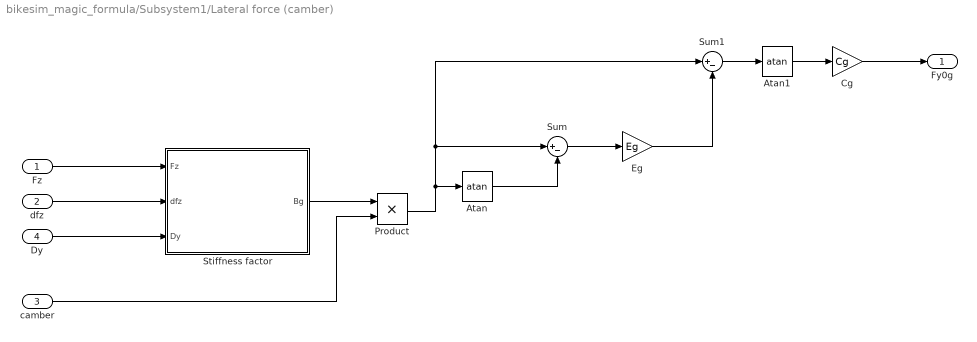
== system bikesim_magic_formula/Subsystem1/Lateral force (camber) ==
  Fz : Inport
  dfz : Inport  Port=2
  camber : Inport  Port=3
  Dy : Inport  Port=4
  Atan : Trigonometry  Operator=atan
  Atan1 : Trigonometry  Operator=atan
  Cg : Gain  Gain=Cg
  Eg : Gain  Gain=Eg
  Product : Product
  Stiffness factor : Subsystem  mask{Cg=Cg, pky6=pky6, pky7=pky7}
      mask prompts: Cg "C_g"; pky6 "p_Ky6"; pky7 "p_Ky7"
      mask TypeOptions Cg: Cg/Gain
  Sum : Sum  Inputs=|+-
  Sum1 : Sum  Inputs=|+-
  Fy0g : Outport
  wires:
  Fz/1 -> Stiffness factor/1(Fz)
  dfz/1 -> Stiffness factor/2(dfz)
  Dy/1 -> Stiffness factor/3(Dy)
  Cg/1 -> Fy0g/1
  Sum1/1 -> Atan1/1
  Product/1 -> Sum1/1, Sum/1, Atan/1
  Atan/1 -> Sum/2
  Atan1/1 -> Cg/1
  Stiffness factor/1(Bg) -> Product/1
  camber/1 -> Product/2
  Sum/1 -> Eg/1
  Eg/1 -> Sum1/2

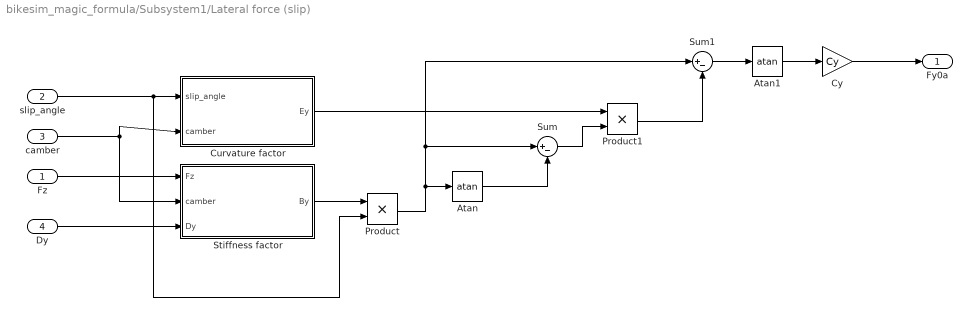
== system bikesim_magic_formula/Subsystem1/Lateral force (slip) ==
  Fz : Inport
  slip_angle : Inport  Port=2
  camber : Inport  Port=3
  Dy : Inport  Port=4
  Atan : Trigonometry  Operator=atan
  Atan1 : Trigonometry  Operator=atan
  Curvature factor : Subsystem  mask{pey1=pey1, pey2=pey2, pey4=pey4}
      mask prompts: pey1 "p_Ey1"; pey2 "p_Ey2"; pey4 "p_Ey4"
      mask Display:
      | port_label('input', 1, '\beta','Interpreter','tex');
      | port_label('input', 2, '\gamma','Interpreter','tex');
      | port_label('output', 1, 'E_y','Interpreter','tex');
  Cy : Gain  Gain=Cy
  Product : Product
  Product1 : Product
  Stiffness factor : Subsystem  mask{Fz0=Fz0, Cy=Cy, pky1=pky1, pky2=pky2, pky3=pky3, pky4=pky4, pky5=pky5}
      mask prompts: Fz0 "F_z0"; Cy "C_y"; pky1 "p_Ky1"; pky2 "p_Ky2"; pky3 "p_Ky3"; pky4 "p_Ky4"; pky5 "p_Ky5"
      mask TypeOptions Fz0: Fz0/Gain | Fz01/Gain
      mask TypeOptions Cy: Cy/Gain
      mask TypeOptions pky1: pky1/Gain
      mask TypeOptions pky2: pky2/Gain
      mask Display:
      | port_label('input', 1, 'F_z','Interpreter','tex');
      | port_label('input', 2, '\gamma','Interpreter','tex');
      | port_label('input', 3, 'D_y','Interpreter','tex');
      | port_label('output', 1, 'B_y','Interpreter','tex');
  Sum : Sum  Inputs=|+-
  Sum1 : Sum  Inputs=|+-
  Fy0a : Outport
  wires:
  Dy/1 -> Stiffness factor/3(Dy)
  Fz/1 -> Stiffness factor/1(Fz)
  camber/1 -> Curvature factor/2(camber), Stiffness factor/2(camber)
  slip_angle/1 -> Curvature factor/1(slip_angle), Product/2
  Stiffness factor/1(By) -> Product/1
  Atan1/1 -> Cy/1
  Sum/1 -> Product1/2
  Product1/1 -> Sum1/2
  Atan/1 -> Sum/2
  Curvature factor/1(Ey) -> Product1/1
  Product/1 -> Sum1/1, Sum/1, Atan/1
  Sum1/1 -> Atan1/1
  Cy/1 -> Fy0a/1

== system bikesim_magic_formula/Subsystem1/Normal force ratio ==
  Fz : Inport
  Divide : Product  Inputs=*/
  Fz0 : Constant  Value=Fz0
  Sum : Sum  Inputs=|+-
  dfz : Outport
  wires:
  Sum/1 -> Divide/1
  Fz0/1 -> Divide/2, Sum/2
  Divide/1 -> dfz/1
  Fz/1 -> Sum/1

== system bikesim_magic_formula/Subsystem1/Peak factor ==
  Fz : Inport
  dfz : Inport  Port=2
  camber : Inport  Port=3
  Divide : Product  Inputs=**/
  Exp : Math
  Polynomial : Polyval  Coefs=[pdy3 0 1]
  pdy1 : Gain  Gain=pdy1
  pdy2 : Gain  Gain=pdy2
  Dy : Outport
  wires:
  Fz/1 -> pdy1/1  "Fz"
  dfz/1 -> pdy2/1  "dfz"
  pdy2/1 -> Exp/1
  Exp/1 -> Divide/2
  pdy1/1 -> Divide/1
  Polynomial/1 -> Divide/3
  camber/1 -> Polynomial/1  "camber"
  Divide/1 -> Dy/1

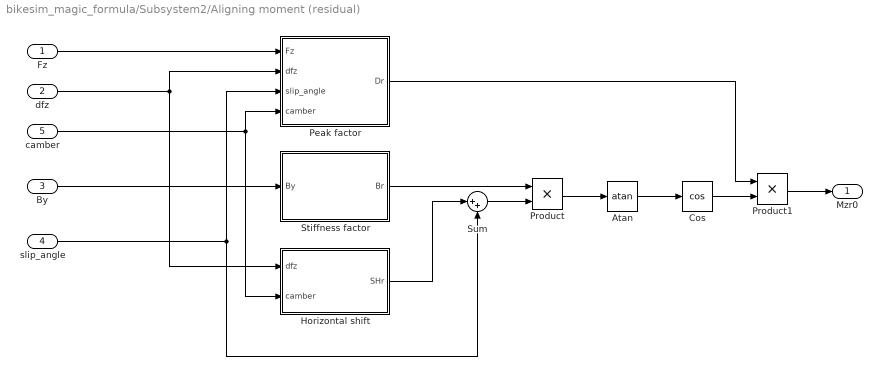
== system bikesim_magic_formula/Subsystem2/Aligning moment (residual) ==
  Fz : Inport
  dfz : Inport  Port=2
  By : Inport  Port=3
  slip_angle : Inport  Port=4
  camber : Inport  Port=5
  Atan : Trigonometry  Operator=atan
  Cos : Trigonometry  Operator=cos
  Horizontal shift : Subsystem  mask{qhz3=qhz3, qhz4=qhz4}
      mask prompts: qhz3 "q_Hz3"; qhz4 "q_Hz4"
      mask Display:
      | port_label('input', 1, 'df_{z}','Interpreter','tex');
      | port_label('input', 2, '\gamma','Interpreter','tex');
      | port_label('output', 1, 'S_{Hr}','Interpreter','tex');
  Peak factor : Subsystem  mask{R0=R0, qdz8=qdz8, qdz9=qdz9, qdz10=qdz10, qdz11=qdz11}
      mask prompts: R0 "R_0"; qdz8 "q_Dz8"; qdz9 "q_Dz9"; qdz10 "q_Dz10"; qdz11 "q_Dz11"
      mask TypeOptions R0: R0/Gain
      mask Display:
      | port_label('input', 1, 'F_z','Interpreter','tex');
      | port_label('input', 2, 'df_z','Interpreter','tex');
      | port_label('input', 3, '\beta','Interpreter','tex');
      | port_label('input', 4, '\gamma','Interpreter','tex');
      | port_label('output', 1, 'D_r','Interpreter','tex');
  Product : Product
  Product1 : Product
  Stiffness factor : Subsystem  mask{Cy=Cy, qbz9=qbz9, qbz10=qbz10}
      mask prompts: Cy "C_y"; qbz9 "q_Bz9"; qbz10 "q_Bz10"
      mask TypeOptions Cy: Cy/Gain
      mask Display:
      | port_label('input', 1, 'B_y','Interpreter','tex');
      | port_label('output', 1, 'B_r','Interpreter','tex');
  Sum : Sum  Inputs=|++
  Mzr0 : Outport
  wires:
  Horizontal shift/1(SHr) -> Sum/1
  slip_angle/1 -> Sum/2, Peak factor/3(slip_angle)
  Sum/1 -> Product/2
  Stiffness factor/1(Br) -> Product/1
  Product/1 -> Atan/1
  Atan/1 -> Cos/1
  Cos/1 -> Product1/2
  Peak factor/1(Dr) -> Product1/1
  Product1/1 -> Mzr0/1
  Fz/1 -> Peak factor/1(Fz)
  dfz/1 -> Peak factor/2(dfz), Horizontal shift/1(dfz)
  camber/1 -> Horizontal shift/2(camber), Peak factor/4(camber)
  By/1 -> Stiffness factor/1(By)

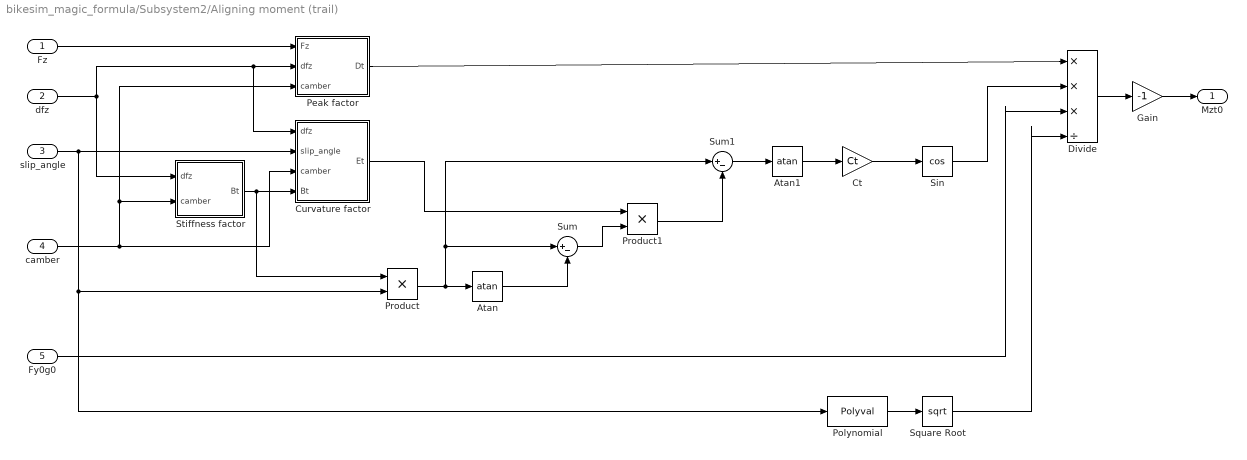
== system bikesim_magic_formula/Subsystem2/Aligning moment (trail) ==
  Fz : Inport
  dfz : Inport  Port=2
  slip_angle : Inport  Port=3
  camber : Inport  Port=4
  Fy0g0 : Inport  Port=5
  Atan : Trigonometry  Operator=atan
  Atan1 : Trigonometry  Operator=atan
  Ct : Gain  Gain=Ct
  Curvature factor : Subsystem  mask{Ct=Ct, qez1=qez1, qez2=qez2, qez5=qez5}
      mask prompts: Ct "C_t"; qez1 "q_Ez1"; qez2 "q_Ez2"; qez5 "q_Ez5"
      mask TypeOptions Ct: Ct/Gain
      mask Display:
      | port_label('input', 1, 'df_z','Interpreter','tex');
      | port_label('input', 2, '\beta','Interpreter','tex');
      | port_label('input', 3, '\gamma','Interpreter','tex');
      | port_label('input', 4, 'B_t','Interpreter','tex');
      | port_label('output', 1, 'E_t','Interpreter','tex');
  Divide : Product  Inputs=***/
  Gain : Gain  Gain=-1
  Peak factor : Subsystem  mask{R0=R0, Fz0=Fz0, qdz1=qdz1, qdz2=qdz2, qdz3=qdz3, qdz4=qdz4}
      mask prompts: R0 "R_0"; Fz0 "F_z0"; qdz1 "q_Dz1"; qdz2 "q_Dz2"; qdz3 "q_Dz3"; qdz4 "q_Dz4"
      mask TypeOptions R0: R0/Gain
      mask TypeOptions Fz0: Fz0/Value
      mask TypeOptions qdz3: qdz3/Gain
      mask Display:
      | port_label('input', 1, 'F_z','Interpreter','tex');
      | port_label('input', 2, 'df_z','Interpreter','tex');
      | port_label('input', 3, '\gamma','Interpreter','tex');
      | port_label('output', 1, 'D_t','Interpreter','tex');
  Polynomial : Polyval  Coefs=[1,0,1]
  Product : Product
  Product1 : Product
  Sin : Trigonometry  Operator=cos
  Square Root : Sqrt
  Stiffness factor : Subsystem  mask{qbz1=qbz1, qbz2=qbz2, qbz5=qbz5, qbz6=qbz6}
      mask prompts: qbz1 "q_Bz1"; qbz2 "q_Bz2"; qbz5 "q_Bz5"; qbz6 "q_Bz6"
      mask TypeOptions qbz5: qbz5/Gain
      mask Display:
      | port_label('input', 1, 'df_{z}','Interpreter','tex');
      | port_label('input', 2, '\gamma','Interpreter','tex');
      | port_label('output', 1, 'B_t','Interpreter','tex');
  Sum : Sum  Inputs=|+-
  Sum1 : Sum  Inputs=|+-
  Mzt0 : Outport
  wires:
  Fz/1 -> Peak factor/1(Fz)
  dfz/1 -> Curvature factor/1(dfz), Peak factor/2(dfz), Stiffness factor/1(dfz)
  camber/1 -> Peak factor/3(camber), Stiffness factor/2(camber), Curvature factor/3(camber)
  slip_angle/1 -> Polynomial/1, Product/2, Curvature factor/2(slip_angle)
  Stiffness factor/1(Bt) -> Product/1, Curvature factor/4(Bt)
  Curvature factor/1(Et) -> Product1/1
  Sum/1 -> Product1/2
  Atan1/1 -> Ct/1
  Product1/1 -> Sum1/2
  Atan/1 -> Sum/2
  Product/1 -> Sum1/1, Sum/1, Atan/1
  Sum1/1 -> Atan1/1
  Ct/1 -> Sin/1
  Sin/1 -> Divide/2
  Peak factor/1(Dt) -> Divide/1
  Fy0g0/1 -> Divide/3
  Polynomial/1 -> Square Root/1
  Square Root/1 -> Divide/4
  Divide/1 -> Gain/1
  Gain/1 -> Mzt0/1

== system bikesim_magic_formula/Subsystem2/Normal force ratio ==
  Fz : Inport
  Divide : Product  Inputs=*/
  Fz0 : Constant  Value=Fz0
  Sum : Sum  Inputs=|+-
  dfz : Outport
  wires:
  Sum/1 -> Divide/1
  Fz0/1 -> Divide/2, Sum/2
  Divide/1 -> dfz/1
  Fz/1 -> Sum/1

== system bikesim_magic_formula/Subsystem2/Peak factor ==
  Fz : Inport
  dfz : Inport  Port=2
  camber : Inport  Port=3
  Divide : Product  Inputs=**/
  Exp : Math
  Polynomial : Polyval  Coefs=[pdy3 0 1]
  pdy1 : Gain  Gain=pdy1
  pdy2 : Gain  Gain=pdy2
  Dy : Outport
  wires:
  Fz/1 -> pdy1/1  "Fz"
  dfz/1 -> pdy2/1  "dfz"
  pdy2/1 -> Exp/1
  Exp/1 -> Divide/2
  pdy1/1 -> Divide/1
  Polynomial/1 -> Divide/3
  camber/1 -> Polynomial/1  "camber"
  Divide/1 -> Dy/1

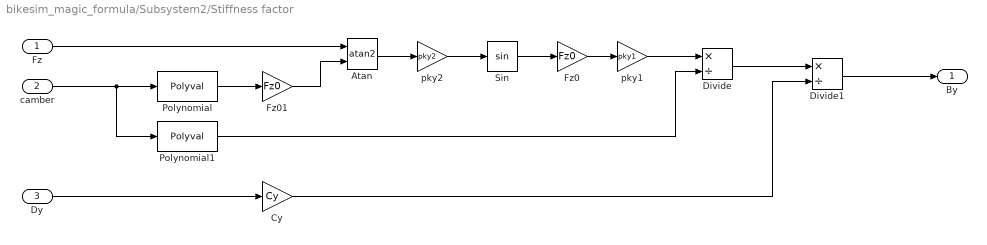
== system bikesim_magic_formula/Subsystem2/Stiffness factor ==
  Fz : Inport
  camber : Inport  Port=2
  Dy : Inport  Port=3
  Atan : Trigonometry  Operator=atan2
  Cy : Gain  Gain=Cy
  Divide : Product  Inputs=*/
  Divide1 : Product  Inputs=*/
  Fz0 : Gain  Gain=Fz0
  Fz01 : Gain  Gain=Fz0
  Polynomial : Polyval  Coefs=[pky4,0,pky3]
  Polynomial1 : Polyval  Coefs=[pky5,0,1]
  Sin : Trigonometry
  pky1 : Gain  Gain=pky1
  pky2 : Gain  Gain=pky2
  By : Outport
  wires:
  Dy/1 -> Cy/1
  Fz0/1 -> pky1/1
  Sin/1 -> Fz0/1
  pky2/1 -> Sin/1
  Atan/1 -> pky2/1
  Fz/1 -> Atan/1
  Fz01/1 -> Atan/2
  Polynomial/1 -> Fz01/1
  camber/1 -> Polynomial1/1, Polynomial/1
  pky1/1 -> Divide/1
  Polynomial1/1 -> Divide/2
  Divide/1 -> Divide1/1
  Cy/1 -> Divide1/2
  Divide1/1 -> By/1

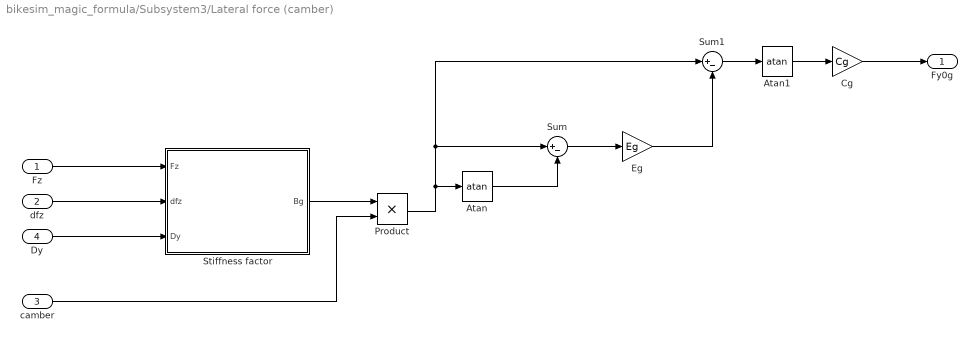
== system bikesim_magic_formula/Subsystem3/Lateral force (camber) ==
  Fz : Inport
  dfz : Inport  Port=2
  camber : Inport  Port=3
  Dy : Inport  Port=4
  Atan : Trigonometry  Operator=atan
  Atan1 : Trigonometry  Operator=atan
  Cg : Gain  Gain=Cg
  Eg : Gain  Gain=Eg
  Product : Product
  Stiffness factor : Subsystem  mask{Cg=Cg, pky6=pky6, pky7=pky7}
      mask prompts: Cg "C_g"; pky6 "p_Ky6"; pky7 "p_Ky7"
      mask TypeOptions Cg: Cg/Gain
  Sum : Sum  Inputs=|+-
  Sum1 : Sum  Inputs=|+-
  Fy0g : Outport
  wires:
  Fz/1 -> Stiffness factor/1(Fz)
  dfz/1 -> Stiffness factor/2(dfz)
  Dy/1 -> Stiffness factor/3(Dy)
  Cg/1 -> Fy0g/1
  Sum1/1 -> Atan1/1
  Product/1 -> Sum1/1, Sum/1, Atan/1
  Atan/1 -> Sum/2
  Atan1/1 -> Cg/1
  Stiffness factor/1(Bg) -> Product/1
  camber/1 -> Product/2
  Sum/1 -> Eg/1
  Eg/1 -> Sum1/2

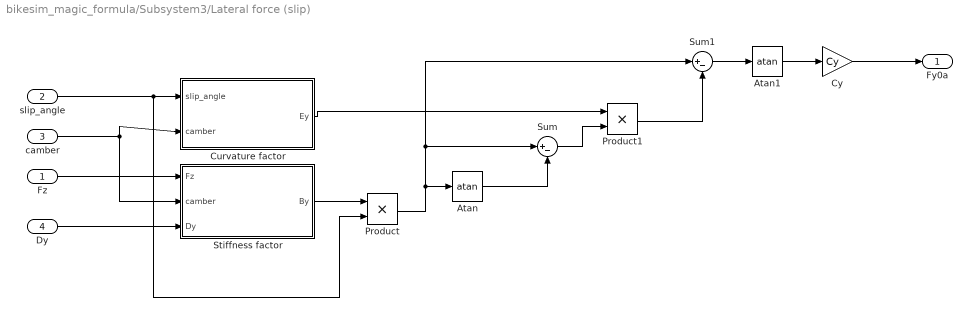
== system bikesim_magic_formula/Subsystem3/Lateral force (slip) ==
  Fz : Inport
  slip_angle : Inport  Port=2
  camber : Inport  Port=3
  Dy : Inport  Port=4
  Atan : Trigonometry  Operator=atan
  Atan1 : Trigonometry  Operator=atan
  Curvature factor : Subsystem  mask{pey1=pey1, pey2=pey2, pey4=pey4}
      mask prompts: pey1 "p_Ey1"; pey2 "p_Ey2"; pey4 "p_Ey4"
      mask Display:
      | port_label('input', 1, '\beta','Interpreter','tex');
      | port_label('input', 2, '\gamma','Interpreter','tex');
      | port_label('output', 1, 'E_y','Interpreter','tex');
  Cy : Gain  Gain=Cy
  Product : Product
  Product1 : Product
  Stiffness factor : Subsystem  mask{Fz0=Fz0, Cy=Cy, pky1=pky1, pky2=pky2, pky3=pky3, pky4=pky4, pky5=pky5}
      mask prompts: Fz0 "F_z0"; Cy "C_y"; pky1 "p_Ky1"; pky2 "p_Ky2"; pky3 "p_Ky3"; pky4 "p_Ky4"; pky5 "p_Ky5"
      mask TypeOptions Fz0: Fz0/Gain | Fz01/Gain
      mask TypeOptions Cy: Cy/Gain
      mask TypeOptions pky1: pky1/Gain
      mask TypeOptions pky2: pky2/Gain
      mask Display:
      | port_label('input', 1, 'F_z','Interpreter','tex');
      | port_label('input', 2, '\gamma','Interpreter','tex');
      | port_label('input', 3, 'D_y','Interpreter','tex');
      | port_label('output', 1, 'B_y','Interpreter','tex');
  Sum : Sum  Inputs=|+-
  Sum1 : Sum  Inputs=|+-
  Fy0a : Outport
  wires:
  Dy/1 -> Stiffness factor/3(Dy)
  Fz/1 -> Stiffness factor/1(Fz)
  camber/1 -> Curvature factor/2(camber), Stiffness factor/2(camber)
  slip_angle/1 -> Curvature factor/1(slip_angle), Product/2
  Stiffness factor/1(By) -> Product/1
  Atan1/1 -> Cy/1
  Sum/1 -> Product1/2
  Product1/1 -> Sum1/2
  Atan/1 -> Sum/2
  Curvature factor/1(Ey) -> Product1/1
  Product/1 -> Sum1/1, Sum/1, Atan/1
  Sum1/1 -> Atan1/1
  Cy/1 -> Fy0a/1

== system bikesim_magic_formula/Subsystem3/Normal force ratio ==
  Fz : Inport
  Divide : Product  Inputs=*/
  Fz0 : Constant  Value=Fz0
  Sum : Sum  Inputs=|+-
  dfz : Outport
  wires:
  Sum/1 -> Divide/1
  Fz0/1 -> Divide/2, Sum/2
  Divide/1 -> dfz/1
  Fz/1 -> Sum/1

== system bikesim_magic_formula/Subsystem3/Peak factor ==
  Fz : Inport
  dfz : Inport  Port=2
  camber : Inport  Port=3
  Divide : Product  Inputs=**/
  Exp : Math
  Polynomial : Polyval  Coefs=[pdy3 0 1]
  pdy1 : Gain  Gain=pdy1
  pdy2 : Gain  Gain=pdy2
  Dy : Outport
  wires:
  Fz/1 -> pdy1/1  "Fz"
  dfz/1 -> pdy2/1  "dfz"
  pdy2/1 -> Exp/1
  Exp/1 -> Divide/2
  pdy1/1 -> Divide/1
  Polynomial/1 -> Divide/3
  camber/1 -> Polynomial/1  "camber"
  Divide/1 -> Dy/1

== system bikesim_magic_formula/Subsystem1/Lateral force (camber)/Stiffness factor ==
  Fz : Inport
  dfz : Inport  Port=2
  Dy : Inport  Port=3
  Cg : Gain  Gain=Cg
  Divide : Product  Inputs=*/
  Polynomial : Polyval  Coefs=[pky7,pky6]
  Product : Product
  Bg : Outport
  wires:
  dfz/1 -> Polynomial/1
  Fz/1 -> Product/1
  Polynomial/1 -> Product/2
  Dy/1 -> Cg/1
  Product/1 -> Divide/1
  Cg/1 -> Divide/2
  Divide/1 -> Bg/1

== system bikesim_magic_formula/Subsystem1/Lateral force (slip)/Curvature factor ==
  slip_angle : Inport
  camber : Inport  Port=2
  Polynomial : Polyval  Coefs=[pey2,0,pey1]
  Polynomial1 : Polyval  Coefs=[pey4,0]
  Product : Product
  Sign : Signum
  Sum : Sum  Inputs=|++
  Ey : Outport
  wires:
  Polynomial1/1 -> Product/1
  Sign/1 -> Product/2
  slip_angle/1 -> Sign/1
  camber/1 -> Polynomial1/1, Polynomial/1
  Product/1 -> Sum/2
  Polynomial/1 -> Sum/1
  Sum/1 -> Ey/1

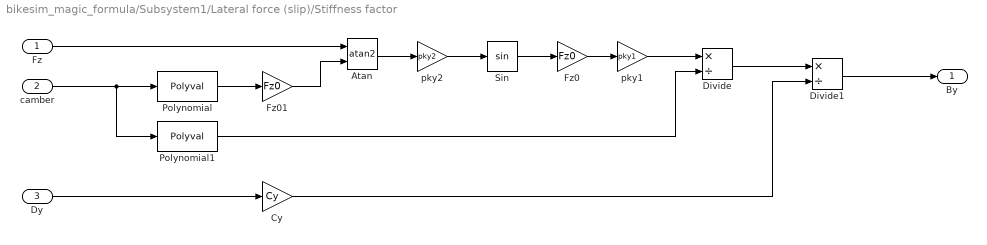
== system bikesim_magic_formula/Subsystem1/Lateral force (slip)/Stiffness factor ==
  Fz : Inport
  camber : Inport  Port=2
  Dy : Inport  Port=3
  Atan : Trigonometry  Operator=atan2
  Cy : Gain  Gain=Cy
  Divide : Product  Inputs=*/
  Divide1 : Product  Inputs=*/
  Fz0 : Gain  Gain=Fz0
  Fz01 : Gain  Gain=Fz0
  Polynomial : Polyval  Coefs=[pky4,0,pky3]
  Polynomial1 : Polyval  Coefs=[pky5,0,1]
  Sin : Trigonometry
  pky1 : Gain  Gain=pky1
  pky2 : Gain  Gain=pky2
  By : Outport
  wires:
  Dy/1 -> Cy/1
  Fz0/1 -> pky1/1
  Sin/1 -> Fz0/1
  pky2/1 -> Sin/1
  Atan/1 -> pky2/1
  Fz/1 -> Atan/1
  Fz01/1 -> Atan/2
  Polynomial/1 -> Fz01/1
  camber/1 -> Polynomial1/1, Polynomial/1
  pky1/1 -> Divide/1
  Polynomial1/1 -> Divide/2
  Divide/1 -> Divide1/1
  Cy/1 -> Divide1/2
  Divide1/1 -> By/1

== system bikesim_magic_formula/Subsystem2/Aligning moment (residual)/Horizontal shift ==
  dfz : Inport
  camber : Inport  Port=2
  Polynomial : Polyval  Coefs=[qhz4,qhz3]
  Product : Product
  SHr : Outport
  wires:
  dfz/1 -> Polynomial/1
  Polynomial/1 -> Product/1
  camber/1 -> Product/2
  Product/1 -> SHr/1

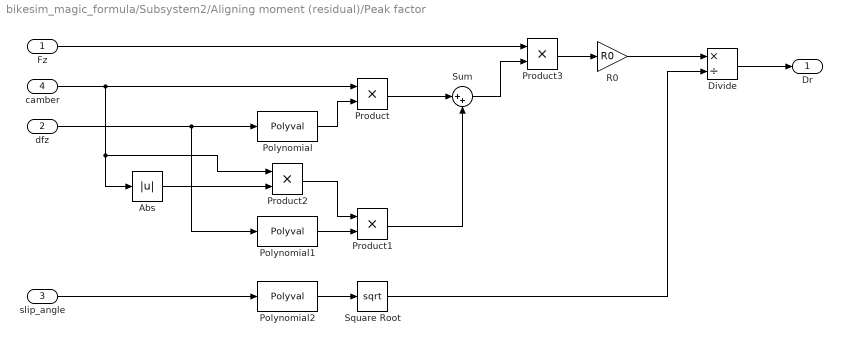
== system bikesim_magic_formula/Subsystem2/Aligning moment (residual)/Peak factor ==
  Fz : Inport
  dfz : Inport  Port=2
  slip_angle : Inport  Port=3
  camber : Inport  Port=4
  Abs : Abs  SaturateOnIntegerOverflow=off
  Divide : Product  Inputs=*/
  Polynomial : Polyval  Coefs=[qdz9,qdz8]
  Polynomial1 : Polyval  Coefs=[qdz11,qdz10]
  Polynomial2 : Polyval  Coefs=[1,0,1]
  Product{,1..3} (4 alike) : Product
  R0 : Gain  Gain=R0
  Square Root : Sqrt
  Sum : Sum  Inputs=|++
  Dr : Outport
  wires:
  Polynomial/1 -> Product/2
  Polynomial1/1 -> Product1/2
  camber/1 -> Abs/1, Product2/1, Product/1
  Abs/1 -> Product2/2
  Product2/1 -> Product1/1
  dfz/1 -> Polynomial1/1, Polynomial/1
  Product/1 -> Sum/1
  Product1/1 -> Sum/2
  Sum/1 -> Product3/2
  Fz/1 -> Product3/1
  Product3/1 -> R0/1
  R0/1 -> Divide/1
  Polynomial2/1 -> Square Root/1
  Square Root/1 -> Divide/2
  slip_angle/1 -> Polynomial2/1
  Divide/1 -> Dr/1

== system bikesim_magic_formula/Subsystem2/Aligning moment (residual)/Stiffness factor ==
  By : Inport
  Cy : Gain  Gain=Cy
  Polynomial : Polyval  Coefs=[qbz10,qbz9]
  Br : Outport
  wires:
  By/1 -> Cy/1
  Cy/1 -> Polynomial/1
  Polynomial/1 -> Br/1

== system bikesim_magic_formula/Subsystem2/Aligning moment (trail)/Curvature factor ==
  dfz : Inport
  slip_angle : Inport  Port=2
  camber : Inport  Port=3
  Bt : Inport  Port=4
  Atan : Trigonometry  Operator=atan
  Ct : Gain  Gain=Ct
  Gain : Gain  Gain=2/pi
  Polynomial : Polyval  Coefs=[qez5,1]
  Polynomial1 : Polyval  Coefs=[qez2,qez1]
  Product : Product
  Product1 : Product
  Product2 : Product
  Et : Outport
  wires:
  Bt/1 -> Ct/1
  Ct/1 -> Product/1
  slip_angle/1 -> Product/2
  Product/1 -> Atan/1
  Atan/1 -> Product1/1
  camber/1 -> Product1/2
  Product1/1 -> Gain/1
  Gain/1 -> Polynomial/1
  dfz/1 -> Polynomial1/1
  Polynomial1/1 -> Product2/1
  Polynomial/1 -> Product2/2
  Product2/1 -> Et/1

== system bikesim_magic_formula/Subsystem2/Aligning moment (trail)/Peak factor ==
  Fz : Inport
  dfz : Inport  Port=2
  camber : Inport  Port=3
  Abs : Abs  SaturateOnIntegerOverflow=off
  Divide : Product  Inputs=*/
  Fz0 : Constant  Value=Fz0
  Polynomial : Polyval  Coefs=[qdz2,qdz1]
  Polynomial1 : Polyval  Coefs=[qdz4 0 1]
  Product : Product  Inputs=3
  R0 : Gain  Gain=R0
  Sum : Sum  Inputs=|++
  qdz3 : Gain  Gain=qdz3
  Dt : Outport
  wires:
  qdz3/1 -> Sum/2
  dfz/1 -> Polynomial/1
  Polynomial1/1 -> Sum/1
  Abs/1 -> qdz3/1
  Product/1 -> Dt/1
  Polynomial/1 -> Product/1
  Sum/1 -> Product/2
  camber/1 -> Abs/1, Polynomial1/1
  Fz/1 -> R0/1
  R0/1 -> Divide/1
  Fz0/1 -> Divide/2
  Divide/1 -> Product/3

== system bikesim_magic_formula/Subsystem2/Aligning moment (trail)/Stiffness factor ==
  dfz : Inport
  camber : Inport  Port=2
  Abs : Abs  SaturateOnIntegerOverflow=off
  Polynomial : Polyval  Coefs=[qbz2,qbz1]
  Polynomial1 : Polyval  Coefs=[qbz6 0 1]
  Product : Product
  Sum : Sum  Inputs=|++
  qbz5 : Gain  Gain=qbz5
  Bt : Outport
  wires:
  dfz/1 -> Polynomial/1
  camber/1 -> Abs/1, Polynomial1/1
  Abs/1 -> qbz5/1
  Polynomial1/1 -> Sum/1
  qbz5/1 -> Sum/2
  Polynomial/1 -> Product/1
  Sum/1 -> Product/2
  Product/1 -> Bt/1

== system bikesim_magic_formula/Subsystem3/Lateral force (camber)/Stiffness factor ==
  Fz : Inport
  dfz : Inport  Port=2
  Dy : Inport  Port=3
  Cg : Gain  Gain=Cg
  Divide : Product  Inputs=*/
  Polynomial : Polyval  Coefs=[pky7,pky6]
  Product : Product
  Bg : Outport
  wires:
  dfz/1 -> Polynomial/1
  Fz/1 -> Product/1
  Polynomial/1 -> Product/2
  Dy/1 -> Cg/1
  Product/1 -> Divide/1
  Cg/1 -> Divide/2
  Divide/1 -> Bg/1

== system bikesim_magic_formula/Subsystem3/Lateral force (slip)/Curvature factor ==
  slip_angle : Inport
  camber : Inport  Port=2
  Polynomial : Polyval  Coefs=[pey2,0,pey1]
  Polynomial1 : Polyval  Coefs=[pey4,0]
  Product : Product
  Sign : Signum
  Sum : Sum  Inputs=|++
  Ey : Outport
  wires:
  Polynomial1/1 -> Product/1
  Sign/1 -> Product/2
  slip_angle/1 -> Sign/1
  camber/1 -> Polynomial1/1, Polynomial/1
  Product/1 -> Sum/2
  Polynomial/1 -> Sum/1
  Sum/1 -> Ey/1
